simulink model "Control_v2"  (R2019b)
settings: Solver=FixedStepAuto  StartTime=0.0  StopTime=10  FixedStep=str2num(Step_size)  RelTol=1e-3
model workspace: external: MATLAB File H:\4-project\matlab\github\Sim-v2\bicopter_sim\Bicopter_DataFile14.m (data not in the file)
values from neighbouring files (symbols this model uses):
  b = [5,1,5,4]    [init_ADRC_val.m]    (also in init_Non_Linear_ADRC_val.m = 0.5*[1,    1, 6,  6]')
  b_sep = gains(5:8)    [get_ADRC_parameters.m]    (also in get_adrc_sep.m = [  2   7    6   7]; get_adrc_sep_kalman.m = [  2   2    6   7])
  C = [eye(4),zeros(4,8)]    [init_ADRC_val.m]
  C_air = 0.0025    [Sim_Script.m]
  d_f_phi = 100    [Sim_Script.m]
  d_f_psi = 25    [Sim_Script.m]
  d_f_theta = 10    [Sim_Script.m]
  d_f_z = 100    [Sim_Script.m]
  eps_sep = 0.7*[1 1 1 1]    [get_ADRC_parameters.m]    (also in get_adrc_sep.m = [0.7 0.3 0.3 0.35]; get_adrc_sep_kalman.m = [0.7 0.7 0.3 0.35])
  epsi = 1.5    [init_Non_Linear_ADRC_val.m]
  euler_source = 1    [Sim_Script.m]
  freq_cut_angvel_phi = 75    [Sim_Script.m]
  freq_cut_angvel_psi = 75    [Sim_Script.m]
  freq_cut_angvel_theta = 50    [Sim_Script.m]
  g = 9.81    [Sim_Script.m]
  K = place(A1,B1,w00(1:8))    [init_ADRC_val.m]
  L = place(A',C',8*w00)'    [init_ADRC_val.m]
  method = STSC_controller    (= 2)    [Sim_Script.m]
  method_angle_plane_sw = plane_sw    (= 2)    [Sim_Script.m]
  mult_obs = 10    [init_Non_Linear_ADRC_val.m]
  Noise_gain = 1    [Sim_Script.m]
  PID_VAL_SEP = init_pid_val_sep()    [Sim_Script.m]
  polarity = [-1;1;1;1]    [Sim_Script.m]
  r = [10,5,10,10]    [init_Non_Linear_ADRC_val.m]
  S_phi = 0.001    [Sim_Script.m]
  S_psi = S_phi    (= 0.001)    [Sim_Script.m]
  S_theta = S_phi    (= 0.001)    [Sim_Script.m]
  State_step = [Z_step;Phi_step;Theta_step;Psi_step]    [req_response.m]
  Step_size = step_size    [Sim_Script.m]
  STSC_VAL = init_STSC_val()    [Sim_Script.m]
  time_delay = 1e-6    (= 1e-06)    [Sim_Script.m]
  V_phi = 0.01    [Sim_Script.m]
  V_psi = 0.01    [Sim_Script.m]
  V_theta = 0.01    [Sim_Script.m]
  wc_sep = gains(1:4)    [get_ADRC_parameters.m]    (also in get_adrc_sep.m = [ 5.54   9   6    3]; get_adrc_sep_kalman.m = [ 5.54   9   6    3])
  wo_sep = ga*wc_sep    [get_ADRC_parameters.m]    (also in get_adrc_sep.m; get_adrc_sep_kalman.m)
undefined symbols (not defined in the file or in its folder): Continuous, magnitude, NLADRC_VAL, sigbuilder_block, smiData, Time, X, Y, Z
libraries: sm_lib x141, nesl_utility x20, simulink x19, fuzblock x3, sharedtransform x1, ctrlSharedLib x1
(part 1 of 7)
settings Model: Creator=HP  LastModifiedBy=HP
settings DataIOCC: SaveFormat=Array  SignalLogging=off  DSMLogging=off  ReturnWorkspaceOutputs=off  OutputSaveName=Pz
settings DiagnosticsConfigSet: SimMechanicsRigidlyBoundBlock=none
settings ExplorerConfigSet: SimMechanicsOpenEditorOnUpdate=off

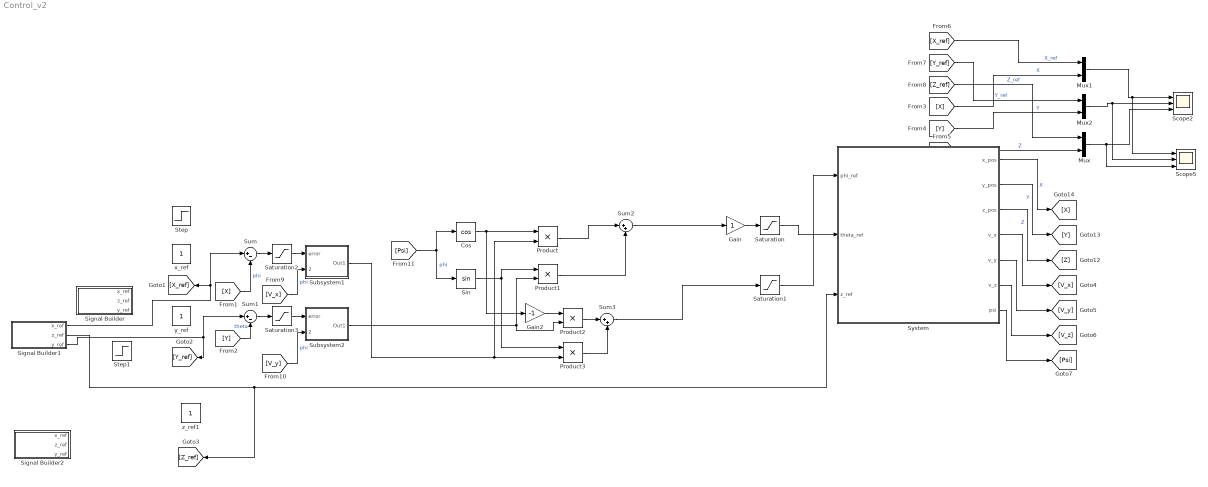
== system Control_v2 ==
  Cos : Trigonometry  Operator=cos
  Gain : Gain
  Gain2 : Gain  Gain=-1
  Mux : Mux  Inputs=2
  Mux1 : Mux  Inputs=2
  Mux2 : Mux  Inputs=2
  Product{,1..3} (4 alike) : Product
  Saturation : Saturate  UpperLimit=0.8  LowerLimit=-0.8
  Saturation1 : Saturate  UpperLimit=0.8  LowerLimit=-0.8
  Saturation2 : Saturate  UpperLimit=3  LowerLimit=-3
  Saturation3 : Saturate  UpperLimit=3  LowerLimit=-3
  Scope2 : Scope  NumInputPorts=3
  Scope5 : Scope  NumInputPorts=3
  Signal Builder : Subsystem  Tag=STV Subsys  LoadFcn=sigbuilder_block('load');  StartFcn=sigbuilder_block('start');  StopFcn=sigbuilder_block('stop');  ClipboardFcn=sigbuilder_block('clipboard');  mask(Sigbuilder block){tuvar=[0:10]}
      mask help: Simulink:masks:SigbuilderBlock_MD
      mask init:
      | if ~strcmp(get_param(bdroot(gcbh),'SimulationStatus'),'stopped') tuvar = sigbuilder_block('maskInit'); end
      settings: CopyFcn=sigbuilder_block('copy');  DeleteFcn=sigbuilder_block('delete');  ModelCloseFcn=sigbuilder_block('modelClose');  PreSaveFcn=sigbuilder_block('preSave');  PauseFcn=sigbuilder_block('pause');  ContinueFcn=sigbuilder_block('continue');  NameChangeFcn=sigbuilder_block('namechange');  OpenFcn=sigbuilder_block('open',[6 30.75 1012.5 481.5 ]);  CloseFcn=sigbuilder_block('close');
      mask Display: plot(0, 0, 100, 100,[2, 2, 32, 32, 2], [68, 8, 8, 68, 68],[32, 2], [38, 38], [32, 19, 2],[53, 60, 44], [32, 17, 17, 2],[16, 16, 31, 31]);txt = getActiveGroup(gcbh);text(2, 100, txt,'verticalAlignment', 'top');
  Signal Builder1 : Subsystem  Tag=STV Subsys  LoadFcn=sigbuilder_block('load');  StartFcn=sigbuilder_block('start');  StopFcn=sigbuilder_block('stop');  ClipboardFcn=sigbuilder_block('clipboard');  mask(Sigbuilder block){tuvar=[0:10]}
      mask help: Simulink:masks:SigbuilderBlock_MD
      mask init:
      | if ~strcmp(get_param(bdroot(gcbh),'SimulationStatus'),'stopped') tuvar = sigbuilder_block('maskInit'); end
      settings: CopyFcn=sigbuilder_block('copy');  DeleteFcn=sigbuilder_block('delete');  ModelCloseFcn=sigbuilder_block('modelClose');  PreSaveFcn=sigbuilder_block('preSave');  PauseFcn=sigbuilder_block('pause');  ContinueFcn=sigbuilder_block('continue');  NameChangeFcn=sigbuilder_block('namechange');  OpenFcn=sigbuilder_block('open',[6 6 1012.5 506.25 ]);  CloseFcn=sigbuilder_block('close');
      mask Display: plot(0, 0, 100, 100,[2, 2, 32, 32, 2], [68, 8, 8, 68, 68],[32, 2], [38, 38], [32, 19, 2],[53, 60, 44], [32, 17, 17, 2],[16, 16, 31, 31]);txt = getActiveGroup(gcbh);text(2, 100, txt,'verticalAlignment', 'top');
  Signal Builder2 : Subsystem  Tag=STV Subsys  LoadFcn=sigbuilder_block('load',[6 6 1012.5 506.25 ]);  StartFcn=sigbuilder_block('start');  StopFcn=sigbuilder_block('stop');  ClipboardFcn=sigbuilder_block('clipboard');  mask(Sigbuilder block){tuvar=[0:10]}
      mask help: Simulink:masks:SigbuilderBlock_MD
      mask init:
      | if ~strcmp(get_param(bdroot(gcbh),'SimulationStatus'),'stopped') tuvar = sigbuilder_block('maskInit'); end
      settings: CopyFcn=sigbuilder_block('copy');  DeleteFcn=sigbuilder_block('delete');  ModelCloseFcn=sigbuilder_block('modelClose');  PreSaveFcn=sigbuilder_block('preSave');  PauseFcn=sigbuilder_block('pause');  ContinueFcn=sigbuilder_block('continue');  NameChangeFcn=sigbuilder_block('namechange');  OpenFcn=sigbuilder_block('open',[-1440 27.75 1440 722.25 ]);  CloseFcn=sigbuilder_block('close');
      mask Display: plot(0, 0, 100, 100,[2, 2, 32, 32, 2], [68, 8, 8, 68, 68],[32, 2], [38, 38], [32, 19, 2],[53, 60, 44], [32, 17, 17, 2],[16, 16, 31, 31]);txt = getActiveGroup(gcbh);text(2, 100, txt,'verticalAlignment', 'top');
  Sin : Trigonometry
  Step : Step  Time=4  SampleTime=0
  Step1 : Step  Time=4  SampleTime=0
  Subsystem1 : Subsystem
  Subsystem2 : Subsystem
  Sum : Sum  Inputs=|+-
  Sum1 : Sum  Inputs=|+-
  Sum2 : Sum  Inputs=|++
  Sum3 : Sum  Inputs=|++
  System : Subsystem
  x_ref : Constant
  y_ref : Constant
  z_ref1 : Constant
  wires:
  System/4(v_x) -> [V_x]
  System/5(v_y) -> [V_y]
  Gain/1 -> Saturation/1
  Sum3/1 -> Saturation1/1
  Sum/1 -> Saturation2/1
  Sum1/1 -> Saturation3/1
  [X] -> Sum/2  "phi"
  [Y] -> Sum1/2  "theta"
  System/1("x_pos ") -> [X]  "X"
  System/2(y_pos) -> [Y]  "Y"
  System/3(z_pos) -> [Z]  "Z"
  [V_x] -> Subsystem1/2(error_dot)  "phi"
  [V_y] -> Subsystem2/2(error_dot)  "phi"
  System/6(v_z) -> [V_z]
  [X_ref] -> Mux1/1  "X_ref"
  [Z_ref] -> Mux/1  "Z_ref"
  [X] -> Mux1/2  "X"
  [Z] -> Mux/2  "Z"
  System/7(psi) -> [Psi]
  [Psi] -> Cos/1, Sin/1  "phi"
  Cos/1 -> Gain2/1, Product/1
  Sin/1 -> Product3/1, Product1/1
  Product/1 -> Sum2/1
  Product1/1 -> Sum2/2
  Subsystem1/1(Out1) -> Product3/2, Product/2
  Subsystem2/1(Out1) -> Product2/2, Product1/2
  Sum2/1 -> Gain/1
  Saturation/1 -> System/2(theta_ref)
  Gain2/1 -> Product2/1
  Product2/1 -> Sum3/1
  Product3/1 -> Sum3/2
  Saturation1/1 -> System/1(phi_ref)
  Saturation2/1 -> Subsystem1/1(error)
  Saturation3/1 -> Subsystem2/1(error)
  Mux1/1 -> Scope5/1, Scope2/1
  Mux/1 -> Scope5/3, Scope2/3
  Mux2/1 -> Scope5/2, Scope2/2
  [Y_ref] -> Mux2/1  "Y_ref"
  [Y] -> Mux2/2  "Y"
  Signal Builder1/1(x_ref) -> [X_ref], Sum/1
  Signal Builder1/2(z_ref) -> [Z_ref], System/3(z_ref)
  Signal Builder1/3(y_ref) -> Sum1/1, [Y_ref]

== system Control_v2/Signal Builder ==
  Demux : Demux  Tag=STV Demux  Outputs=3
  FromWs : FromWorkspace  Tag=STV FromWs  VariableName=tuvar  SampleTime=0
      SigBuilderData=|
      | common.afterFinalStr = 'Extrapolate'
      | common.sampleTime = 0
      | dataSet.timeRange = [0 25]
      | dataSet.name = 'Group 1'
      | sbobj.Groups.Name = 'Group 1'
      | sbobj.Groups.Signals(1).Name = 'x_ref'
      | sbobj.Groups.Signals(1).XData = [0 6.12 6.12 12.78 12.78 19.32 19.32 25]
      | sbobj.Groups.Signals(1).YData = [0 0 2 2 -1 -1 2 2]
      | sbobj.Groups.Signals(2).Name = 'z_ref'
      | sbobj.Groups.Signals(2).XData = [0 6.12 12.78 12.78 19.32 19.32 25]
      | sbobj.Groups.Signals(2).YData = [1 1 1 5 5 2 2]
      | sbobj.Groups.Signals(3).Name = 'y_ref'
      | sbobj.Groups.Signals(3).XData = [0 6.12 6.12 12.78 12.78 19.32 19.32 25]
      | sbobj.Groups.Signals(3).YData = [0 0 -2 -2 1 1 -3 -3]
      | sbobj.Groups.TimeRange = [0 25]
  x_ref : Outport  Tag=STV Outport
  z_ref : Outport  Tag=STV Outport  Port=2
  y_ref : Outport  Tag=STV Outport  Port=3
  wires:
  FromWs/1 -> Demux/1
  Demux/1 -> x_ref/1
  Demux/2 -> z_ref/1
  Demux/3 -> y_ref/1

== system Control_v2/Signal Builder1 ==
  Demux : Demux  Tag=STV Demux  Outputs=3
  FromWs : FromWorkspace  Tag=STV FromWs  VariableName=tuvar  SampleTime=0
      SigBuilderData=|
      | common.afterFinalStr = 'Extrapolate'
      | common.sampleTime = 0
      | dataSet.timeRange = [0 25]
      | dataSet.name = 'Group 1'
      | sbobj.Groups.Name = 'Group 1'
      | sbobj.Groups.Signals(1).Name = 'x_ref'
      | sbobj.Groups.Signals(1).XData = [0 3 3 12.78 12.78 19.32 19.32 25]
      | sbobj.Groups.Signals(1).YData = [0 0 10 10 -1 -1 10 10]
      | sbobj.Groups.Signals(2).Name = 'z_ref'
      | sbobj.Groups.Signals(2).XData = [0 6.12 12.78 12.78 19.32 19.32 25]
      | sbobj.Groups.Signals(2).YData = [1 1 1 5 5 2 2]
      | sbobj.Groups.Signals(3).Name = 'y_ref'
      | sbobj.Groups.Signals(3).XData = [0 3 3 12.78 12.78 19.32 19.32 25]
      | sbobj.Groups.Signals(3).YData = [0 0 -10 -10 10 10 -10 -10]
      | sbobj.Groups.TimeRange = [0 25]
  x_ref : Outport  Tag=STV Outport
  z_ref : Outport  Tag=STV Outport  Port=2
  y_ref : Outport  Tag=STV Outport  Port=3
  wires:
  FromWs/1 -> Demux/1
  Demux/1 -> x_ref/1
  Demux/2 -> z_ref/1
  Demux/3 -> y_ref/1

== system Control_v2/Signal Builder2 ==
  Demux : Demux  Tag=STV Demux  Outputs=3
  FromWs : FromWorkspace  Tag=STV FromWs  VariableName=tuvar  SampleTime=0
      SigBuilderData=|
      | common.afterFinalStr = 'Extrapolate'
      | common.sampleTime = 0
      | dataSet.timeRange = [0 25]
      | dataSet.name = 'Group 1'
      | sbobj.Groups.Name = 'Group 1'
      | sbobj.Groups.Signals(1).Name = 'x_ref'
      | sbobj.Groups.Signals(1).XData = [0 3 3 12.78 12.78 19.32 19.32 25]
      | sbobj.Groups.Signals(1).YData = [0 0 10 10 -1 -1 10 10]
      | sbobj.Groups.Signals(2).Name = 'z_ref'
      | sbobj.Groups.Signals(2).XData = [0 3 3 12.78 19.32 19.32 25]
      | sbobj.Groups.Signals(2).YData = [0 0 10 10 5 2 2]
      | sbobj.Groups.Signals(3).Name = 'y_ref'
      | sbobj.Groups.Signals(3).XData = [0 3 3 12.78 19.32 19.32 25]
      | sbobj.Groups.Signals(3).YData = [0 0 10 10 10 -10 -10]
      | sbobj.Groups.TimeRange = [0 25]
  x_ref : Outport  Tag=STV Outport
  z_ref : Outport  Tag=STV Outport  Port=2
  y_ref : Outport  Tag=STV Outport  Port=3
  wires:
  FromWs/1 -> Demux/1
  Demux/1 -> x_ref/1
  Demux/2 -> z_ref/1
  Demux/3 -> y_ref/1

== system Control_v2/Subsystem1 ==
  error : Inport
  error_dot : Inport  Port=2
  Gain : Gain  Gain=0.005
  Integrator Limited : Integrator  LimitOutput=on  UpperSaturationLimit=1  LowerSaturationLimit=-1
  Sum2 : Sum  Inputs=|++-
  Transfer Fcn : TransferFcn  Denominator=[1 1]
  x_d : Gain  Gain=0.2
  x_p : Gain  Gain=0.14
  Out1 : Outport
  wires:
  x_p/1 -> Sum2/1
  error/1 -> Gain/1, x_p/1
  Sum2/1 -> Out1/1
  Gain/1 -> Integrator Limited/1
  error_dot/1 -> x_d/1
  x_d/1 -> Sum2/3

== system Control_v2/Subsystem2 ==
  error : Inport
  error_dot : Inport  Port=2
  Sum2 : Sum  Inputs=|+-
  y_d : Gain  Gain=0.2
  y_p : Gain  Gain=0.15
  Out1 : Outport
  wires:
  y_d/1 -> Sum2/2
  y_p/1 -> Sum2/1
  error_dot/1 -> y_d/1
  error/1 -> y_p/1
  Sum2/1 -> Out1/1

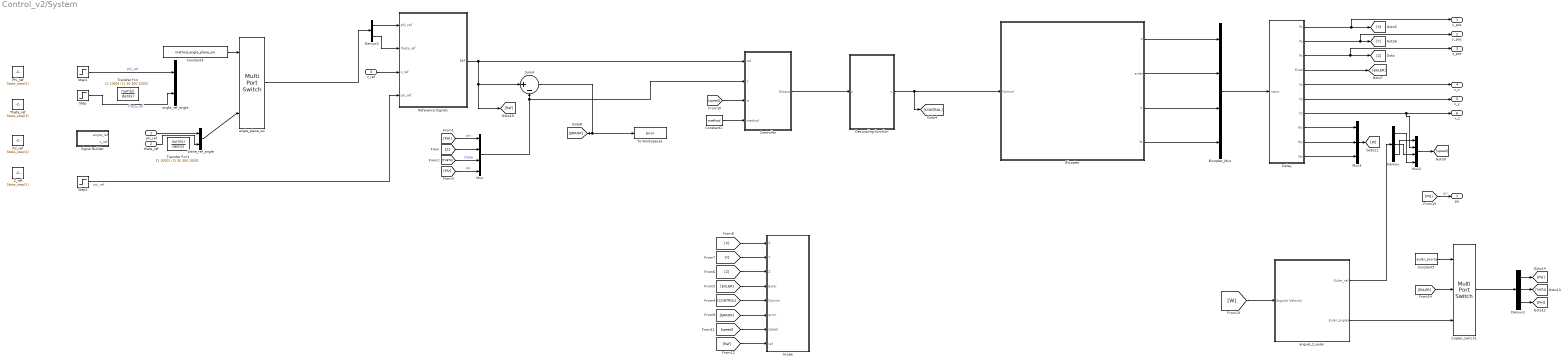
== system Control_v2/System ==
  note: psi_ref
  phi_ref : Inport
  theta_ref : Inport  Port=2
  z_ref : Inport  Port=3
  Bicopter : Subsystem
      mask Display: image('H:\4-project\matlab\Final_Sim\bicopter_sim\Bicopter_photo.PNG'); % Use "Edit Image" on toolstrip to change.
  Bicopter_Mux : Mux
  Constant1 : Constant  Value=method
  Constant3 : Constant  Value=method_angle_plane_sw
  Constant5 : Constant  Value=euler_source
  Controller : Subsystem
  Copter_switch1 : MultiPortSwitch  Inputs=2
  Decoupling function : MATLAB Function  TreatAsAtomicUnit=on
  Delay : Subsystem
  Demux : Demux  Outputs=3
  Demux1 : Demux  Outputs=3
  Demux2 : Demux  Outputs=2
  Mux : Mux
  Mux2 : Mux
  Mux3 : Mux  Inputs=3
  Phi_ref : Constant  Value=State_step(2)
  Psi_ref : Constant  Value=State_step(4)
  Reference Signals : Subsystem
  Scope : Subsystem
  Signal Builder : Subsystem  Tag=STV Subsys  LoadFcn=sigbuilder_block('load');  StartFcn=sigbuilder_block('start');  StopFcn=sigbuilder_block('stop');  ClipboardFcn=sigbuilder_block('clipboard');  mask(Sigbuilder block){tuvar=[0:10]}
      mask help: Simulink:masks:SigbuilderBlock_MD
      mask init:
      | if ~strcmp(get_param(bdroot(gcbh),'SimulationStatus'),'stopped') tuvar = sigbuilder_block('maskInit'); end
      settings: CopyFcn=sigbuilder_block('copy');  DeleteFcn=sigbuilder_block('delete');  ModelCloseFcn=sigbuilder_block('modelClose');  PreSaveFcn=sigbuilder_block('preSave');  PauseFcn=sigbuilder_block('pause');  ContinueFcn=sigbuilder_block('continue');  NameChangeFcn=sigbuilder_block('namechange');  OpenFcn=sigbuilder_block('open',[0.75 265.5 1021.5 480 ]);  CloseFcn=sigbuilder_block('close');
      mask Display: plot(0, 0, 100, 100,[2, 2, 32, 32, 2], [68, 8, 8, 68, 68],[32, 2], [38, 38], [32, 19, 2],[53, 60, 44], [32, 17, 17, 2],[16, 16, 31, 31]);txt = getActiveGroup(gcbh);text(2, 100, txt,'verticalAlignment', 'top');
  Step : Step  Time=4  After=0.5  SampleTime=0
  Step1 : Step  Time=4  After=0  SampleTime=0
  Step2 : Step  Time=4  After=0  SampleTime=0
  Sum4 : Sum  Inputs=|+-
  Theta_ref : Constant  Value=State_step(3)
  To Workspace1 : ToWorkspace  VariableName=Error  SampleTime=-1
  Transfer Fcn : TransferFcn  Numerator=[1 1000]  Denominator=[1 30 300 1000]
  Transfer Fcn1 : TransferFcn  Numerator=[1 1000]  Denominator=[1 30 300 1000]
  Z_ref : Constant  Value=State_step(1)
  angle_plane_sw : MultiPortSwitch  Inputs=2
  angle_ref_angle : Mux  Inputs=2
  angvel_2_euler : Subsystem
  plane_ref_angle : Mux  Inputs=2
  "x_pos " : Outport
  y_pos : Outport  Port=2
  z_pos : Outport  Port=3
  v_x : Outport  Port=4
  v_y : Outport  Port=5
  v_z : Outport  Port=6
  psi : Outport  Port=7
  wires:
  Demux/1 -> Mux2/4
  Delay/9(Wy) -> Mux3/2
  Mux2/1 -> [speed]
  Decoupling function/1(y) -> Bicopter/1("Control "), [CONTROL]
  Controller/1(Output) -> Decoupling function/1(u)
  [speed] -> Scope/7(speed)
  [THETA] -> Mux/3  "theta"
  [CONTROL] -> Scope/5("Control ")
  Delay/7(Vz) -> Mux2/2, v_z/1
  Mux3/1 -> [W]
  Demux/3 -> Mux2/1
  Delay/3(Pz) -> z_pos/1, [Z]
  Demux1/3 -> [PHI]
  Delay/4(Euler) -> [EULER]
  [PHI] -> Mux/1  "phi"
  [Y] -> Scope/2(Y)
  Demux1/2 -> [THETA]
  Delay/5(Vx) -> v_x/1
  [X] -> Scope/1(X)
  Demux/2 -> Mux2/3
  Constant1/1 -> Controller/4(method)
  Bicopter/1(P) -> Bicopter_Mux/1
  Bicopter/3(V) -> Bicopter_Mux/3
  [Z] -> Mux/2
  Delay/2(Py) -> [Y], y_pos/1
  Delay/6(Vy) -> v_y/1
  [ERROR] -> Scope/6(error)
  [EULER] -> Scope/4(Euler)
  Delay/10(Wz) -> Mux3/3
  [speed] -> Controller/3(w)
  Sum4/1 -> To Workspace1/1, [ERROR]
  Delay/1(Px) -> [X], "x_pos "/1
  Demux1/1 -> [PSI]
  Bicopter/4(W) -> Bicopter_Mux/4
  [Ref] -> Scope/8(ref)
  [Z] -> Scope/3(Z)
  Mux/1 -> Controller/2(y), Sum4/2
  [EULER] -> Copter_switch1/2
  Reference Signals/1(REF) -> Controller/1(ref), [Ref], Sum4/1
  Delay/8(Wx) -> Mux3/1
  Constant5/1 -> Copter_switch1/1
  Bicopter/2(euler) -> Bicopter_Mux/2
  Copter_switch1/1 -> Demux1/1
  phi_ref/1 -> plane_ref_angle/1
  angle_plane_sw/1 -> Demux2/1
  Demux2/1 -> Reference Signals/1(phi_ref)
  Demux2/2 -> Reference Signals/2(theta_ref)
  Constant3/1 -> angle_plane_sw/1
  [PSI] -> Mux/4  "psi"
  Step1/1 -> angle_ref_angle/1  "phi_ref"
  z_ref/1 -> Reference Signals/3(z_ref)
  Bicopter_Mux/1 -> Delay/1(input)
  angvel_2_euler/2(Euler_angles) -> Copter_switch1/3
  [W] -> angvel_2_euler/1(Angular Velocity)
  angvel_2_euler/1(Euler_vel) -> Demux/1
  Step2/1 -> Reference Signals/4(psi_ref)
  [PSI] -> psi/1  "psi"
  theta_ref/1 -> plane_ref_angle/2
  Step/1 -> angle_ref_angle/2  "theta_ref"
  plane_ref_angle/1 -> angle_plane_sw/3
